simulink model "simPropelerTestbench"  (R2023b)
settings: Solver=VariableStepAuto  StartTime=0.0  StopTime=10.0  RelTol=1e-3
undefined symbols (not defined in the file or in its folder): uavParam
libraries: simulink x1
settings Model: Creator=jjha  LastModifiedBy=jjha

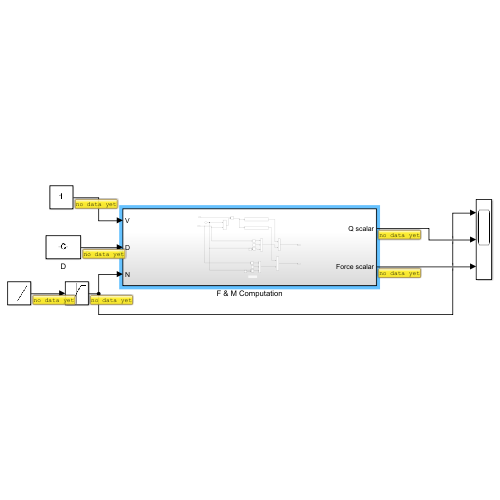
[thumbnail: Simulink's stored preview of the top-level diagram]
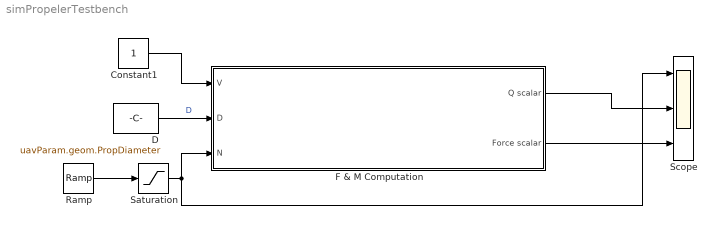
== system simPropelerTestbench ==
  Constant1 : Constant
  D : Constant  Value=uavParam.geom.PropDiameter
  F & M Computation : Subsystem
  Ramp : simulink/Sources/Ramp  slope=15  start=0  InitialOutput=0
  Saturation : Saturate  UpperLimit=500  LowerLimit=16
  Scope : Scope  NumInputPorts=3
  wires:
  F & M Computation/1(Q scalar) -> Scope/2
  F & M Computation/2(Force scalar) -> Scope/3
  Constant1/1 -> F & M Computation/1(V)
  D/1 -> F & M Computation/2(D)  "D"
  Ramp/1 -> Saturation/1
  Saturation/1 -> Scope/1, F & M Computation/3(N)

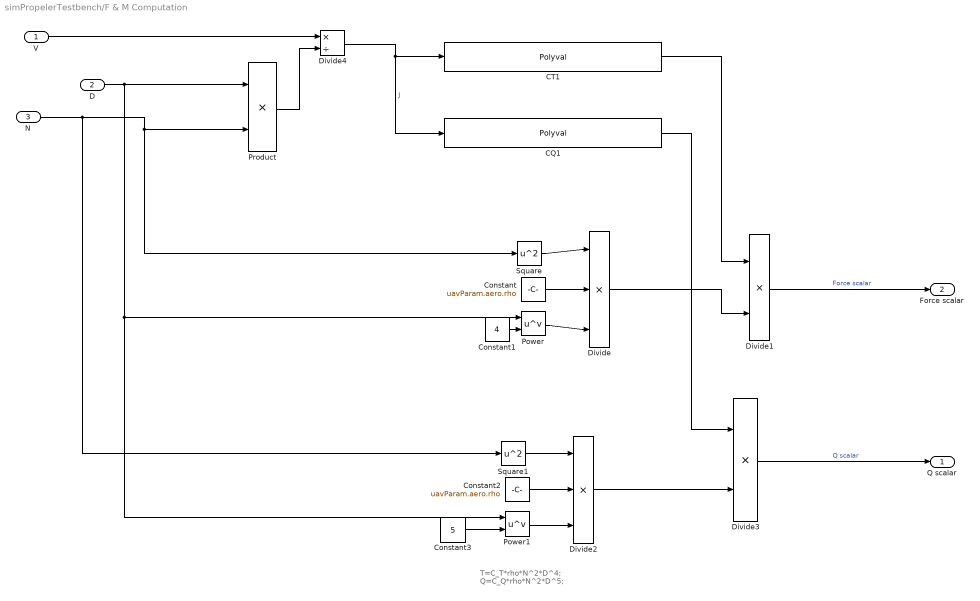
== system simPropelerTestbench/F & M Computation ==
  note: T=C_T*rho*N^2*D^4;
      | Q=C_Q*rho*N^2*D^5;
  V : Inport
  D : Inport  Port=2
  N : Inport  Port=3
  CQ1 : Polyval  Coefs=[0.04280,-0.05046,0.005711,-0.003293, 0.007048]
  CT1 : Polyval  Coefs=[0.03338, -0.1265,-0.1210,0.1142]
  Constant : Constant  Value=uavParam.aero.rho
  Constant1 : Constant  Value=4
  Constant2 : Constant  Value=uavParam.aero.rho
  Constant3 : Constant  Value=5
  Divide : Product  Inputs=***
  Divide1 : Product  Inputs=**
  Divide2 : Product  Inputs=***
  Divide3 : Product  Inputs=**
  Divide4 : Product  Inputs=*/
  Power : Math  Operator=pow
  Power1 : Math  Operator=pow
  Product : Product
  Square : Math  Operator=square
  Square1 : Math  Operator=square
  Q scalar : Outport
  Force scalar : Outport  Port=2
  wires:
  Divide4/1 -> CQ1/1, CT1/1  "J"
  Product/1 -> Divide4/2
  CT1/1 -> Divide1/1
  Divide2/1 -> Divide3/2
  CQ1/1 -> Divide3/1
  Divide3/1 -> Q scalar/1  "Q scalar"
  Divide/1 -> Divide1/2
  Divide1/1 -> Force scalar/1  "Force scalar"
  V/1 -> Divide4/1
  Power/1 -> Divide/3
  Constant/1 -> Divide/2
  Constant3/1 -> Power1/2
  Square/1 -> Divide/1
  Power1/1 -> Divide2/3
  N/1 -> Square/1, Product/2, Square1/1
  D/1 -> Power/1, Power1/1, Product/1
  Constant1/1 -> Power/2
  Square1/1 -> Divide2/1
  Constant2/1 -> Divide2/2
